simulink model "AeroPendulum"  (R2019a)
settings: Solver=ode5  StartTime=0.0  StopTime=inf  FixedStep=Ts  RelTol=1e-3  EnableMultiTasking=on
InitFcn:
  | Ts=0.025;
  | MAX = 110;
  | MIN = 0;
undefined symbols (not defined in the file or in its folder): Serial_Port, Standard_Devices
libraries: simulink x4, sldrtlib x3
settings Model: SimulationMode=external  ExtModeTrigDuration=10000  ExtModeTrigDurationFloating=10000  Creator=HADI  LastModifiedBy=Mashroti
settings DataIOCC: LimitDataPoints=on  SaveFormat=Array  ReturnWorkspaceOutputs=off
settings OptimizationCC: ExpressionDepthLimit=2147483647
settings DebuggingCC: UnderspecifiedInitializationDetection=Classic  MergeDetectMultiDrivingBlocksExec=none  SolverPrmCheckMsg=warning  StateNameClashWarn=warning  SFUnexpectedBacktrackingDiag=warning  SFNoUnconditionalDefaultTransitionDiag=warning  SFExecutionAtInitializationDiag=none  ArithmeticOperatorsInVariantConditions=warning
settings ModelReferenceCC: PropagateSignalLabelsOutOfModel=off
settings SFSimCC: SimUseLocalCustomCode=off
settings RTWCC: SystemTargetFile=sldrt.tlc  TemplateMakefile=sldrt.tmf  Description=Simulink Desktop Real-Time  RTWUseLocalCustomCode=off  RTWCompilerOptimization=on
settings CodeAppCC: MaxIdLength=95  StateflowObjectComments=on
settings SimulinkDesktopRealTimeCC: TargetPreCompLibLocation=C:\Program Files\Polyspace\R2019a\toolbox\sldrt\lib\win64  TargetLangStandard=C89/C90 (ANSI)  SupportVariableSizeSignals=off  PreserveStateflowLocalDataDimensions=off
settings ConfigComp: CovMetricSettings=dw  CovHtmlReporting=on  CovSaveCumulativeToWorkspaceVar=on  CovSaveSingleToWorkspaceVar=on  CovExternalEMLEnable=off

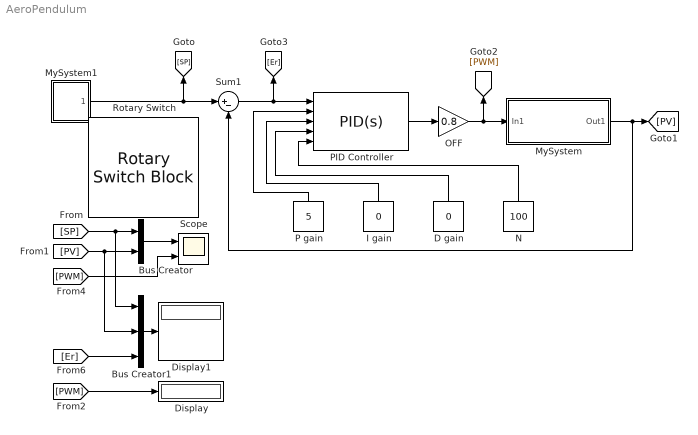
== system AeroPendulum ==
  Bus Creator : BusCreator  Inputs=2
  Bus Creator1 : BusCreator  Inputs=3
  D gain : Constant  Value=0  SampleTime=Ts
  Display : Display
  Display1 : Display
  I gain : Constant  Value=0  SampleTime=Ts
  MySystem : Subsystem  Description=sasd
  MySystem1 : Subsystem  Description=sasd
  N : Constant  Value=100  SampleTime=Ts
  OFF : Gain  Gain=0.8  OutDataTypeStr=double
  P gain : Constant  Value=5  SampleTime=Ts
  PID Controller : simulink/Continuous/PID Controller  Controller=PID  Form=Parallel  TimeDomain=Continuous-time  SampleTime=-1  IntegratorMethod=Forward Euler  FilterMethod=Forward Euler  ControllerParametersSource=external  P=5  I=1  D=1  UseFilter=on  N=1  TunerSelectOption=Transfer Function Based (PID Tuner App)  InitialConditionSource=internal  InitialConditionForIntegrator=0  InitialConditionForFilter=0  DifferentiatorICPrevScaledInput=0  ExternalReset=none  TrackingMode=off  Kt=1  LimitOutput=on  UpperSaturationLimit=MAX  LowerSaturationLimit=MIN  LinearizeAsGain=off  AntiWindupMode=none  Kb=1  POutMin=MIN  POutMax=MAX  IOutMin=MIN  IOutMax=MAX  DOutMin=MIN  DOutMax=MAX  NOutMin=MIN  NOutMax=MAX  SumOutMin=MIN  SumOutMax=MAX  SaturationOutMin=MIN  SaturationOutMax=MAX  PParamMin=[]  PParamMax=[]  IParamMin=[]  IParamMax=[]  DParamMin=[]  DParamMax=[]  NParamMin=[]  NParamMax=[]  KbParamMin=[]  KbParamMax=[]  KtParamMin=[]  KtParamMax=[]  KbOutMin=[]  KbOutMax=[]  KtOutMin=[]  KtOutMax=[]  IntegratorOutMin=[]  IntegratorOutMax=[]  FilterOutMin=[]  FilterOutMax=[]  SumI1OutMin=[]  SumI1OutMax=[]  SumI2OutMin=[]  SumI2OutMax=[]  SumI3OutMin=[]  SumI3OutMax=[]  SumI4OutMin=[]  SumI4OutMax=[]  SumDOutMin=[]  SumDOutMax=[]  DifferentiatorOutMin=[]  DifferentiatorOutMax=[]  FilterDiffOutCoefMin=[]  FilterDiffOutCoefMax=[]  ReciprocalOutMin=[]  ReciprocalOutMax=[]  SumDenOutMin=[]  SumDenOutMax=[]  SumNumOutMin=[]  SumNumOutMax=[]  DivideOutMin=[]  DivideOutMax=[]  IntegratorContinuousStateAttributes=''  IntegratorStateMustResolveToSignalObject=off  IntegratorRTWStateStorageClass=Auto  FilterContinuousStateAttributes=''  FilterStateMustResolveToSignalObject=off  FilterRTWStateStorageClass=Auto  ParallelPVariant=ExternalParameters  IdealPVariant=Disabled  IVariant=ExternalParameters  DVariant=ExternalParameters  IntegratorVariant=Continuous  SatVariant=Enabled  AWVariant=Passthrough  PCopyVariant=Disabled  TRVariant=Disabled  FdbkBlocksVariant=Forward  IdealPFdbkVariant=Disabled  SatFdbkVariant=Disabled  DerivativeFilterVariant=ContFilter  NVariant=ExternalParameters  NCopyVariant=Disabled  FilterICVariant=InternalICsFilter  IntegratorICVariant=InternalICs  ExternalResetVariant=Disabled  TRSumVariant=Passthrough  SumFdbkVariant=Disabled  SumVariant=Sum_PID
      settings: LockScale=on
  Rotary Switch : RotarySwitchBlock  LabelPosition=Hide
      settings: Values={{'sin', 'step', 'ramp'}, [0 1 2]}
  Scope : Scope  NumInputPorts=2
  Sum1 : Sum  Inputs=|+-
  wires:
  Bus Creator/1 -> Scope/1
  MySystem/1(Out1) -> Sum1/2, [PV]
  Bus Creator1/1 -> Display1/1
  MySystem1/1(Out1) -> Sum1/1, [SP]
  PID Controller/1 -> OFF/1
  Sum1/1 -> PID Controller/1, [Er]
  OFF/1 -> [PWM], MySystem/1(In1)
  [PWM] -> Scope/2
  [SP] -> Bus Creator1/1, Bus Creator/1
  [PV] -> Bus Creator1/2, Bus Creator/2
  [PWM] -> Display/1
  [Er] -> Bus Creator1/3
  P gain/1 -> PID Controller/2
  I gain/1 -> PID Controller/3
  D gain/1 -> PID Controller/4
  N/1 -> PID Controller/5

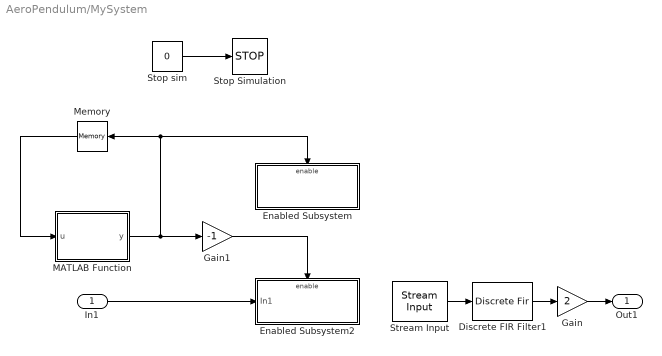
== system AeroPendulum/MySystem ==
  In1 : Inport
  Discrete FIR Filter1 : DiscreteFir  FilterStructure=Direct form symmetric  SampleTime=Ts
  Enabled Subsystem : Subsystem  TreatAsAtomicUnit=on
  Enabled Subsystem2 : Subsystem  TreatAsAtomicUnit=on
  Gain : Gain  Gain=2
  Gain1 : Gain  Gain=-1
  MATLAB Function : MATLAB Function  TreatAsAtomicUnit=on
  Memory : Memory  InitialCondition=20
  Stop Simulation : Stop
  Stop sim : Constant  Value=0
  Stream Input : sldrtlib/Stream Input  SampleTime=Ts  MaxMissedTicks=10  ShowMissedTicks=off  YieldWhenWaiting=off  DrvName=Standard_Devices/Serial_Port  DrvAddress=5  DrvOptions=[115200 8 0 0 0 0 0 0]  DataTypes='double'  FormatString='%e'  Terminator={'\r', '\n'}  ShowReady=off  ShowError=off
      settings: AttributesFormatString=Serial Port [5]  SourceProductName=Simulink Desktop Real-Time  SourceProductBaseCode=WT
  Out1 : Outport
  wires:
  Stop sim/1 -> Stop Simulation/1
  MATLAB Function/1(y) -> Memory/1, Enabled Subsystem/Enable, Gain1/1
  Gain1/1 -> Enabled Subsystem2/Enable
  In1/1 -> Enabled Subsystem2/1(In1)
  Stream Input/1 -> Discrete FIR Filter1/1
  Memory/1 -> MATLAB Function/1(u)
  Discrete FIR Filter1/1 -> Gain/1
  Gain/1 -> Out1/1

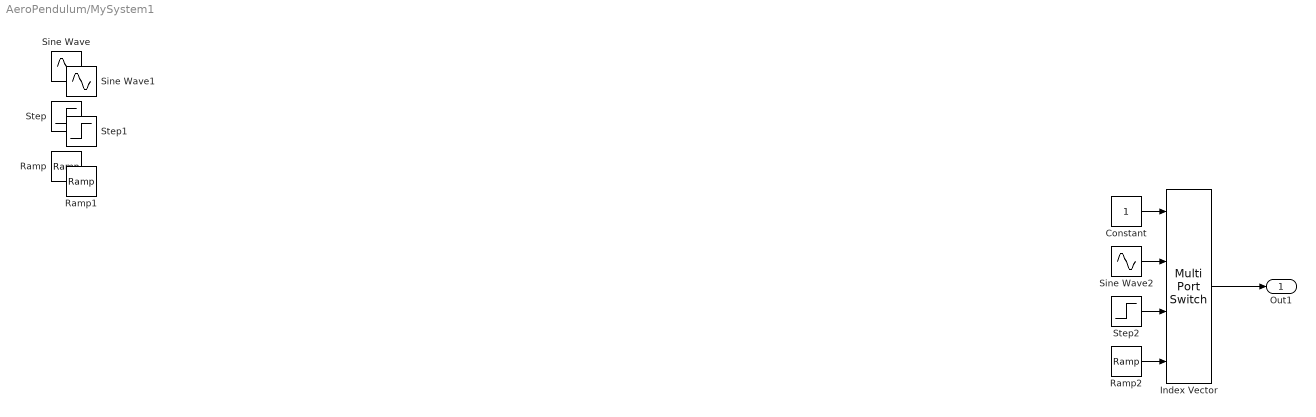
== system AeroPendulum/MySystem1 ==
  Constant : Constant
  Index Vector : MultiPortSwitch  DataPortOrder=Zero-based contiguous  zeroidx=on
  Ramp : simulink/Sources/Ramp  slope=1  start=0  InitialOutput=0
  Ramp1 : simulink/Sources/Ramp  slope=1  start=0  InitialOutput=0
  Ramp2 : simulink/Sources/Ramp  slope=1  start=0  InitialOutput=0
  Sine Wave : Sin  Amplitude=10  Bias=45  Frequency=0.5  SampleTime=0
  Sine Wave1 : Sin  Amplitude=10  Bias=45  Frequency=0.5  SampleTime=0
  Sine Wave2 : Sin  Amplitude=10  Bias=45  Frequency=0.5  SampleTime=0
  Step : Step  SampleTime=0
  Step1 : Step  SampleTime=0
  Step2 : Step  SampleTime=0
  Out1 : Outport
  wires:
  Ramp2/1 -> Index Vector/4
  Step2/1 -> Index Vector/3
  Sine Wave2/1 -> Index Vector/2
  Index Vector/1 -> Out1/1
  Constant/1 -> Index Vector/1

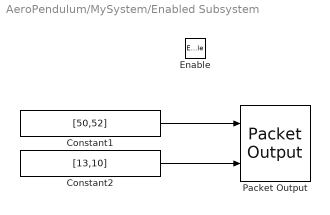
== system AeroPendulum/MySystem/Enabled Subsystem ==
  Enable : EnablePort
  Constant1 : Constant  Value=[50,52]
  Constant2 : Constant  Value=[13,10]
  Packet Output : sldrtlib/Packet Output  SampleTime=Ts  MaxMissedTicks=10  ShowMissedTicks=off  YieldWhenWaiting=on  DrvName=Standard_Devices/Serial_Port  DrvAddress=5  DrvOptions=[115200 8 0 0 0 0 0 0]  PacketSize=4  DataTypes={'2*int8', '2*int8'}  ShowReady=off  ShowError=off  PacketID=1  ByteOrder=1  InitialValue=[]  FinalValue=[]
      settings: AttributesFormatString=Serial Port [5]  SourceProductName=Simulink Desktop Real-Time
  wires:
  Constant1/1 -> Packet Output/1
  Constant2/1 -> Packet Output/2

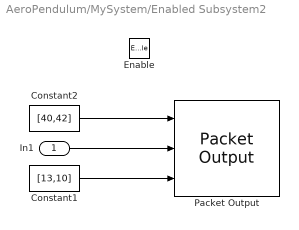
== system AeroPendulum/MySystem/Enabled Subsystem2 ==
  In1 : Inport
  Enable : EnablePort
  Constant1 : Constant  Value=[13,10]
  Constant2 : Constant  Value=[40,42]
  Packet Output : sldrtlib/Packet Output  SampleTime=Ts  MaxMissedTicks=10  ShowMissedTicks=off  YieldWhenWaiting=off  DrvName=Standard_Devices/Serial_Port  DrvAddress=5  DrvOptions=[115200 8 0 0 0 0 0 0]  PacketSize=12  DataTypes={'2*int8','1*double', '2*int8'}  ShowReady=off  ShowError=off  PacketID=1  ByteOrder=1  InitialValue=[]  FinalValue=[]
      settings: AttributesFormatString=Serial Port [5]  SourceProductName=Simulink Desktop Real-Time
  wires:
  In1/1 -> Packet Output/2
  Constant1/1 -> Packet Output/3
  Constant2/1 -> Packet Output/1

== matlab function AeroPendulum/MySystem/MATLAB Function ==
  data: u input; y output
function y = fcn(u)
%#codegen
y=u;
if u==20
    y=-20;
elseif u==-20
    y=20;
end
